simulink model "CHANGE_crazyflie_simulation_paper"  (R2019a)
settings: Solver=FixedStepAuto  StartTime=0.0  StopTime=50  FixedStep=Ts  RelTol=1e-3
values from neighbouring files (symbols this model uses):
  b = 0.033    [CHANGE_set_params_paper.m]    (also in plot_responses_paper.m = 0.25; set_params.m; set_params_paper.m)
  D_0 = 4/(Ts^2) + 4*zeta*omega_n/Ts + omega_n^2    (= 1011376)    [CHANGE_set_params_paper.m]    (also in set_params.m = 1057500; set_params_paper.m = 1057500)
  D_1 = -8/(Ts^2) + 2*omega_n^2    (= -1999872)    [CHANGE_set_params_paper.m]    (also in set_params.m = -1995000; set_params_paper.m = -1995000)
  D_2 = 4/(Ts^2) - 4*zeta*omega_n/Ts + omega_n^2    (= 988752)    [CHANGE_set_params_paper.m]    (also in set_params.m = 947500; set_params_paper.m = 947500)
  g = 9.81    [CHANGE_set_params_paper.m]    (also in set_params.m; set_params_paper.m)
  I_CF_1 = [16.823890  -1.224320  -0.716891 ... (first row only)    [CHANGE_set_params_paper.m]    (also in set_params.m; set_params_paper.m)
  I_CF_1_inv = inv(I_CF_1)    [CHANGE_set_params_paper.m]    (also in set_params.m; set_params_paper.m)
  I_rzz = 9.3e-9    (= 9.3e-09)    [CHANGE_set_params_paper.m]    (also in set_params.m; set_params_paper.m)
  k_f = 1.6e-4    (= 0.00016)    [CHANGE_set_params_paper.m]    (also in set_params.m; set_params_paper.m)
  k_m = 1e-6    (= 1e-06)    [CHANGE_set_params_paper.m]    (also in set_params.m; set_params_paper.m)
  kx = 10.25e-4    (= 0.001025)    [CHANGE_set_params_paper.m]    (also in set_params.m; set_params_paper.m)
  ky = 10.25e-4    (= 0.001025)    [CHANGE_set_params_paper.m]    (also in set_params.m; set_params_paper.m)
  kz = 7.553e-4    (= 0.0007553)    [CHANGE_set_params_paper.m]    (also in set_params.m; set_params_paper.m)
  l = 0.033    [CHANGE_set_params_paper.m]    (also in set_params.m; set_params_paper.m)
  m_CF = 0.028    [CHANGE_set_params_paper.m]    (also in set_params.m; set_params_paper.m)
  N_0 = omega_n^2    (= 64)    [CHANGE_set_params_paper.m]    (also in set_params.m = 2500; set_params_paper.m = 2500)
  N_1 = 2*omega_n^2    (= 128)    [CHANGE_set_params_paper.m]    (also in set_params.m = 5000; set_params_paper.m = 5000)
  N_2 = omega_n^2    (= 64)    [CHANGE_set_params_paper.m]    (also in set_params.m = 2500; set_params_paper.m = 2500)
  omegaR_init = [1; 1; 1; 1]*200    [CHANGE_set_params_paper.m]    (also in set_params.m; set_params_paper.m)
  T = 0.061658    [CHANGE_set_params_paper.m]    (also in inner_pd.m = 0.0666666666667; outer_pd_cs.m = 0.0666666666667; set_params.m = 0.0617; set_params_paper.m)
  T_init = m_CF*0.1    (= 0.0028)    [CHANGE_set_params_paper.m]    (also in set_params.m; set_params_paper.m)
  Ts = 1/500    (= 0.002)    [CHANGE_set_params_paper.m]    (also in inner_pd.m = 0.01; outer_pd_cs.m = 0.01; set_params.m; set_params_paper.m)
undefined symbols (not defined in the file or in its folder): DiscIntNeverNeededParam, sigbuilder_block
libraries: sharedutil x4, simulink x2
(part 2 of 2)

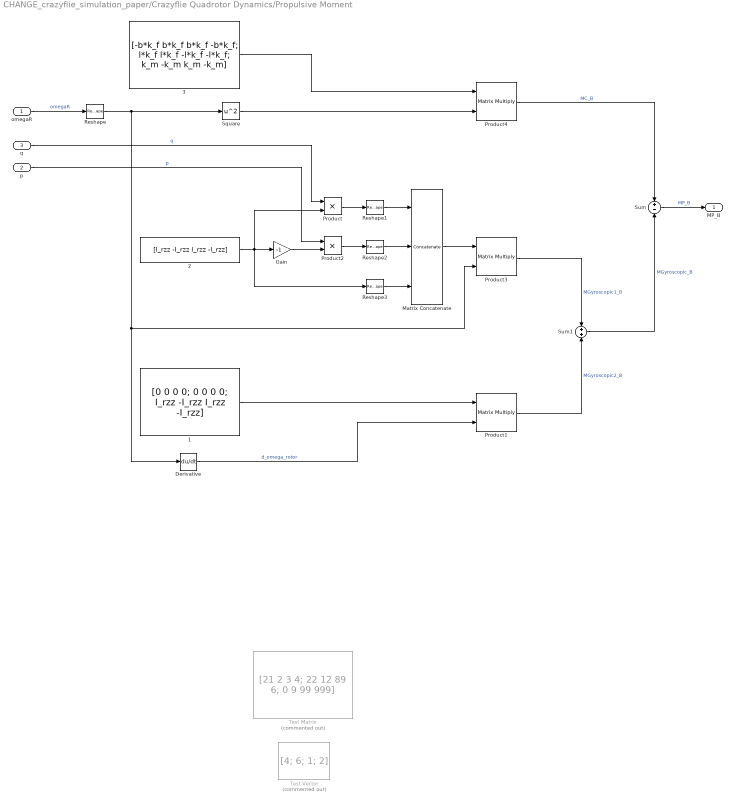
== system CHANGE_crazyflie_simulation_paper/Crazyflie Quadrotor Dynamics/Propulsive Moment ==
  omegaR : Inport
  p : Inport  Port=2
  q : Inport  Port=3
  "  1" : Constant  Value=[0 0 0 0; 0 0 0 0; I_rzz -I_rzz I_rzz -I_rzz]
  "  2" : Constant  Value=[I_rzz -I_rzz I_rzz -I_rzz]
  "  3" : Constant  Value=[-b*k_f b*k_f b*k_f -b*k_f; l*k_f l*k_f -l*k_f -l*k_f; k_m -k_m k_m -k_m]
  "  Test Matrix" : Constant  Commented=on  Value=[21 2 3 4; 22 12 89 6; 0 9 99 999]
  Derivative : Derivative
  Gain : Gain  Gain=-1
  Matrix Concatenate : Concatenate  NumInputs=3  Mode=Multidimensional array
  Product : Product
  Product1 : Product  Multiplication=Matrix(*)
  Product2 : Product
  Product3 : Product  Multiplication=Matrix(*)
  Product4 : Product  Multiplication=Matrix(*)
  Reshape : Reshape  OutputDimensionality=Column vector (2-D)
  Reshape1 : Reshape  OutputDimensionality=Row vector (2-D)
  Reshape2 : Reshape  OutputDimensionality=Row vector (2-D)
  Reshape3 : Reshape  OutputDimensionality=Row vector (2-D)
  Square : Math  Operator=square  SaturateOnIntegerOverflow=on
  Sum : Sum  Inputs=+-
  Sum1 : Sum
  Test Vector : Constant  Commented=on  Value=[4; 6; 1; 2]
  MP_B : Outport
  wires:
  Matrix Concatenate/1 -> Product3/1
  "  3"/1 -> Product4/1
  q/1 -> Product/1  "q"
  Gain/1 -> Product2/2
  Product1/1 -> Sum1/2  "MGyroscopic2_B"
  Derivative/1 -> Product1/2  "d_omega_rotor"
  "  1"/1 -> Product1/1
  Product3/1 -> Sum1/1  "MGyroscopic1_B"
  p/1 -> Product2/1  "p"
  "  2"/1 -> Product/2, Gain/1, Reshape3/1
  Product2/1 -> Reshape2/1
  Product/1 -> Reshape1/1
  Sum1/1 -> Sum/2  "MGyroscopic_B"
  Sum/1 -> MP_B/1  "MP_B"
  Product4/1 -> Sum/1  "MC_B"
  omegaR/1 -> Reshape/1  "omegaR"
  Reshape1/1 -> Matrix Concatenate/1
  Reshape2/1 -> Matrix Concatenate/2
  Reshape3/1 -> Matrix Concatenate/3
  Reshape/1 -> Square/1, Product3/2, Derivative/1
  Square/1 -> Product4/2

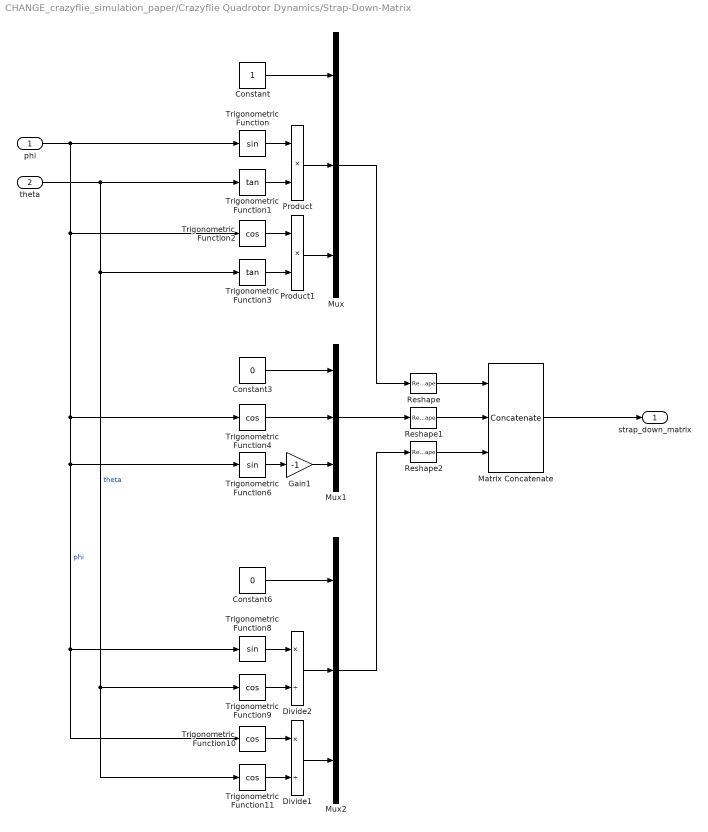
== system CHANGE_crazyflie_simulation_paper/Crazyflie Quadrotor Dynamics/Strap-Down-Matrix ==
  phi : Inport
  theta : Inport  Port=2
  Constant : Constant
  Constant3 : Constant  Value=0
  Constant6 : Constant  Value=0
  Divide1 : Product  Inputs=*/
  Divide2 : Product  Inputs=*/
  Gain1 : Gain  Gain=-1
  Matrix Concatenate : Concatenate  NumInputs=3  Mode=Multidimensional array
  Mux : Mux  Inputs=3
  Mux1 : Mux  Inputs=3
  Mux2 : Mux  Inputs=3
  Product : Product
  Product1 : Product
  Reshape : Reshape  OutputDimensionality=Row vector (2-D)
  Reshape1 : Reshape  OutputDimensionality=Row vector (2-D)
  Reshape2 : Reshape  OutputDimensionality=Row vector (2-D)
  Trigonometric Function : Trigonometry
  Trigonometric Function1 : Trigonometry  Operator=tan
  Trigonometric Function{2,4,9..11} (5 alike) : Trigonometry  Operator=cos
  Trigonometric Function3 : Trigonometry  Operator=tan
  Trigonometric Function6 : Trigonometry
  Trigonometric Function8 : Trigonometry
  strap_down_matrix : Outport
  wires:
  Gain1/1 -> Mux1/3
  Matrix Concatenate/1 -> strap_down_matrix/1
  Mux/1 -> Reshape/1
  Product1/1 -> Mux/3
  Reshape1/1 -> Matrix Concatenate/2
  Constant6/1 -> Mux2/1
  Reshape/1 -> Matrix Concatenate/1
  Constant3/1 -> Mux1/1
  Trigonometric Function4/1 -> Mux1/2
  Trigonometric Function/1 -> Product/1
  Reshape2/1 -> Matrix Concatenate/3
  theta/1 -> Trigonometric Function3/1, Trigonometric Function11/1, Trigonometric Function9/1, Trigonometric Function1/1  "theta"
  Trigonometric Function3/1 -> Product1/2
  Trigonometric Function2/1 -> Product1/1
  Product/1 -> Mux/2
  Divide1/1 -> Mux2/3
  Trigonometric Function9/1 -> Divide2/2
  Trigonometric Function6/1 -> Gain1/1
  Mux2/1 -> Reshape2/1
  Trigonometric Function8/1 -> Divide2/1
  Trigonometric Function1/1 -> Product/2
  Mux1/1 -> Reshape1/1
  Trigonometric Function10/1 -> Divide1/1
  Trigonometric Function11/1 -> Divide1/2
  Divide2/1 -> Mux2/2
  Constant/1 -> Mux/1
  phi/1 -> Trigonometric Function10/1, Trigonometric Function8/1, Trigonometric Function6/1, Trigonometric Function4/1, Trigonometric Function2/1, Trigonometric Function/1  "phi"

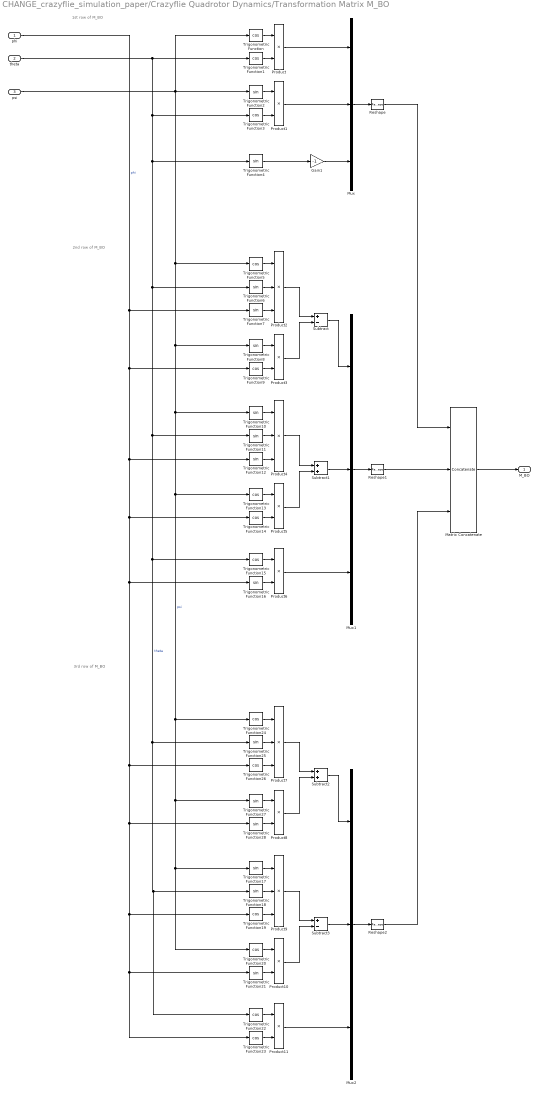
== system CHANGE_crazyflie_simulation_paper/Crazyflie Quadrotor Dynamics/Transformation Matrix M_BO ==
  note: 3rd row of M_BO
  note: 2nd row of M_BO
  note: 1st row of M_BO
  phi : Inport
  theta : Inport  Port=2
  psi : Inport  Port=3
  Gain1 : Gain  Gain=-1
  Matrix Concatenate : Concatenate  NumInputs=3  Mode=Multidimensional array
  Mux : Mux  Inputs=3
  Mux1 : Mux  Inputs=3
  Mux2 : Mux  Inputs=3
  Product{,1,3,5..6,8,10..11} (8 alike) : Product
  Product{2,4,7,9} (4 alike) : Product  Inputs=3
  Reshape : Reshape  OutputDimensionality=Row vector (2-D)
  Reshape1 : Reshape  OutputDimensionality=Row vector (2-D)
  Reshape2 : Reshape  OutputDimensionality=Row vector (2-D)
  Subtract : Sum  Inputs=+-
  Subtract1 : Sum
  Subtract2 : Sum
  Subtract3 : Sum  Inputs=+-
  Trigonometric Function{,1,3,5,9,13..15,19..20,22..24,26} (14 alike) : Trigonometry  Operator=cos
  Trigonometric Function{2,4,6..8,10..12,16..18,21,25,27..28} (15 alike) : Trigonometry
  M_BO : Outport
  wires:
  Gain1/1 -> Mux/3
  Trigonometric Function/1 -> Product/1
  Trigonometric Function1/1 -> Product/2
  psi/1 -> Trigonometric Function20/1, Trigonometric Function17/1, Trigonometric Function27/1, Trigonometric Function24/1, Trigonometric Function13/1, Trigonometric Function10/1, Trigonometric Function8/1, Trigonometric Function5/1, Trigonometric Function/1, Trigonometric Function2/1  "psi"
  Trigonometric Function3/1 -> Product1/2
  Trigonometric Function2/1 -> Product1/1
  Product/1 -> Mux/1
  Product1/1 -> Mux/2
  Trigonometric Function4/1 -> Gain1/1
  Mux/1 -> Reshape/1
  Reshape/1 -> Matrix Concatenate/1
  Trigonometric Function5/1 -> Product2/1
  Trigonometric Function6/1 -> Product2/2
  theta/1 -> Trigonometric Function22/1, Trigonometric Function18/1, Trigonometric Function25/1, Trigonometric Function15/1, Trigonometric Function11/1, Trigonometric Function6/1, Trigonometric Function4/1, Trigonometric Function3/1, Trigonometric Function1/1  "theta"
  Trigonometric Function7/1 -> Product2/3
  phi/1 -> Trigonometric Function23/1, Trigonometric Function21/1, Trigonometric Function19/1, Trigonometric Function28/1, Trigonometric Function26/1, Trigonometric Function16/1, Trigonometric Function14/1, Trigonometric Function12/1, Trigonometric Function9/1, Trigonometric Function7/1  "phi"
  Trigonometric Function8/1 -> Product3/1
  Trigonometric Function9/1 -> Product3/2
  Product2/1 -> Subtract/1
  Product3/1 -> Subtract/2
  Product5/1 -> Subtract1/2
  Product4/1 -> Subtract1/1
  Trigonometric Function14/1 -> Product5/2
  Trigonometric Function13/1 -> Product5/1
  Trigonometric Function12/1 -> Product4/3
  Trigonometric Function11/1 -> Product4/2
  Trigonometric Function10/1 -> Product4/1
  Trigonometric Function16/1 -> Product6/2
  Trigonometric Function15/1 -> Product6/1
  Subtract/1 -> Mux1/1
  Product6/1 -> Mux1/3
  Subtract1/1 -> Mux1/2
  Mux1/1 -> Reshape1/1
  Reshape1/1 -> Matrix Concatenate/2
  Reshape2/1 -> Matrix Concatenate/3
  Mux2/1 -> Reshape2/1
  Subtract3/1 -> Mux2/2
  Product11/1 -> Mux2/3
  Subtract2/1 -> Mux2/1
  Trigonometric Function22/1 -> Product11/1
  Trigonometric Function23/1 -> Product11/2
  Trigonometric Function17/1 -> Product9/1
  Trigonometric Function18/1 -> Product9/2
  Trigonometric Function19/1 -> Product9/3
  Trigonometric Function20/1 -> Product10/1
  Trigonometric Function21/1 -> Product10/2
  Product9/1 -> Subtract3/1
  Product10/1 -> Subtract3/2
  Product8/1 -> Subtract2/2
  Product7/1 -> Subtract2/1
  Trigonometric Function28/1 -> Product8/2
  Trigonometric Function27/1 -> Product8/1
  Trigonometric Function26/1 -> Product7/3
  Trigonometric Function25/1 -> Product7/2
  Trigonometric Function24/1 -> Product7/1
  Matrix Concatenate/1 -> M_BO/1

== system CHANGE_crazyflie_simulation_paper/Crazyflie Quadrotor Dynamics1/Aerodynamic Force ==
  V_B : Inport
  Demux : Demux  Outputs=3
  Gain : Gain  Gain=-kx
  Gain1 : Gain  Gain=-ky
  Gain2 : Gain  Gain=-kz
  Mux1 : Mux  Inputs=3
  Reshape : Reshape  OutputDimensionality=Column vector (2-D)
  FA_B : Outport
  wires:
  Reshape/1 -> FA_B/1  "FA_B"
  Demux/1 -> Gain/1  "v_B"
  Demux/3 -> Gain2/1  "w_B"
  V_B/1 -> Demux/1
  Demux/2 -> Gain1/1  "u_B"
  Gain/1 -> Mux1/1
  Gain1/1 -> Mux1/2
  Mux1/1 -> Reshape/1
  Gain2/1 -> Mux1/3

== system CHANGE_crazyflie_simulation_paper/Crazyflie Quadrotor Dynamics1/Cross Product Custom ==
  A : Inport
  B : Inport  Port=2
  A1 : InportShadow
  B1 : InportShadow  Port=2
  Subsystem : sharedutil/3x3 Cross Product/Subsystem  SystemSampleTime=-1
      settings: SourceProductName=Aerospace Blockset  SourceProductBaseCode=AE
  Subsystem1 : sharedutil/3x3 Cross Product/Subsystem1  SystemSampleTime=-1
      settings: SourceProductName=Aerospace Blockset  SourceProductBaseCode=AE
  Sum3 : Sum  Inputs=+|-  SaturateOnIntegerOverflow=on  InputSameDT=on  OutDataTypeStr=Inherit: Same as first input
  C : Outport
  wires:
  Subsystem/1 -> Sum3/1
  B1/1 -> Subsystem1/2
  Sum3/1 -> C/1
  B/1 -> Subsystem/2
  Subsystem1/1 -> Sum3/2
  A/1 -> Subsystem/1
  A1/1 -> Subsystem1/1

== system CHANGE_crazyflie_simulation_paper/Crazyflie Quadrotor Dynamics1/Gravitational Force  ==
  Product : Product
  Reshape : Reshape  OutputDimensionality=Column vector (2-D)
  g_acc : Constant  Value=[0; 0; g]
  m_CF : Constant  Value=m_CF
  FG_O : Outport
  wires:
  Reshape/1 -> FG_O/1  "FG_O"
  Product/1 -> Reshape/1
  g_acc/1 -> Product/1
  m_CF/1 -> Product/2

== system CHANGE_crazyflie_simulation_paper/Crazyflie Quadrotor Dynamics1/Propulsive Force ==
  omegaR : Inport
  Constant : Constant  Value=0
  Demux1 : Demux
  Gain4 : Gain  Gain=-k_f
  Matrix Sum2 : Sum  Inputs=++++
  Mux : Mux  Inputs=3
  Reshape : Reshape  OutputDimensionality=Column vector (2-D)
  FP_B : Outport
  wires:
  Constant/1 -> Mux/1, Mux/2
  Reshape/1 -> FP_B/1  "FP_B"
  Demux1/3 -> Matrix Sum2/3  "omegaR_3"
  Demux1/1 -> Matrix Sum2/1  "omegaR_1"
  Demux1/4 -> Matrix Sum2/4  "omegaR_4"
  Mux/1 -> Reshape/1
  Matrix Sum2/1 -> Gain4/1
  omegaR/1 -> Demux1/1
  Demux1/2 -> Matrix Sum2/2  "omegaR_2"
  Gain4/1 -> Mux/3

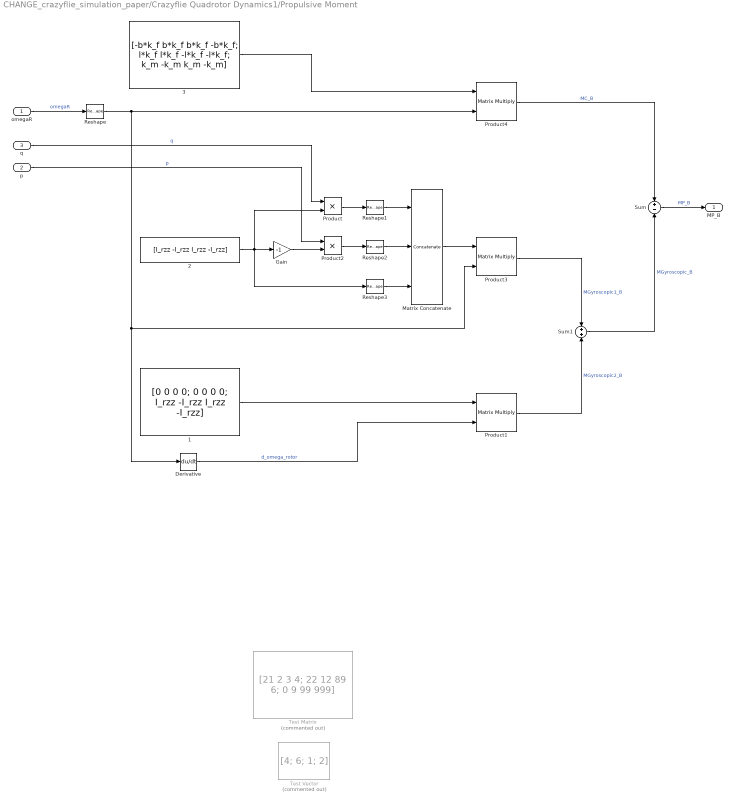
== system CHANGE_crazyflie_simulation_paper/Crazyflie Quadrotor Dynamics1/Propulsive Moment ==
  omegaR : Inport
  p : Inport  Port=2
  q : Inport  Port=3
  "  1" : Constant  Value=[0 0 0 0; 0 0 0 0; I_rzz -I_rzz I_rzz -I_rzz]
  "  2" : Constant  Value=[I_rzz -I_rzz I_rzz -I_rzz]
  "  3" : Constant  Value=[-b*k_f b*k_f b*k_f -b*k_f; l*k_f l*k_f -l*k_f -l*k_f; k_m -k_m k_m -k_m]
  "  Test Matrix" : Constant  Commented=on  Value=[21 2 3 4; 22 12 89 6; 0 9 99 999]
  Derivative : Derivative
  Gain : Gain  Gain=-1
  Matrix Concatenate : Concatenate  NumInputs=3  Mode=Multidimensional array
  Product : Product
  Product1 : Product  Multiplication=Matrix(*)
  Product2 : Product
  Product3 : Product  Multiplication=Matrix(*)
  Product4 : Product  Multiplication=Matrix(*)
  Reshape : Reshape  OutputDimensionality=Column vector (2-D)
  Reshape1 : Reshape  OutputDimensionality=Row vector (2-D)
  Reshape2 : Reshape  OutputDimensionality=Row vector (2-D)
  Reshape3 : Reshape  OutputDimensionality=Row vector (2-D)
  Sum : Sum  Inputs=+-
  Sum1 : Sum
  Test Vector : Constant  Commented=on  Value=[4; 6; 1; 2]
  MP_B : Outport
  wires:
  Matrix Concatenate/1 -> Product3/1
  "  3"/1 -> Product4/1
  Reshape/1 -> Product3/2, Derivative/1, Product4/2
  q/1 -> Product/1  "q"
  Gain/1 -> Product2/2
  Product1/1 -> Sum1/2  "MGyroscopic2_B"
  Derivative/1 -> Product1/2  "d_omega_rotor"
  "  1"/1 -> Product1/1
  Product3/1 -> Sum1/1  "MGyroscopic1_B"
  p/1 -> Product2/1  "p"
  "  2"/1 -> Product/2, Gain/1, Reshape3/1
  Product2/1 -> Reshape2/1
  Product/1 -> Reshape1/1
  Sum1/1 -> Sum/2  "MGyroscopic_B"
  Sum/1 -> MP_B/1  "MP_B"
  Product4/1 -> Sum/1  "MC_B"
  omegaR/1 -> Reshape/1  "omegaR"
  Reshape1/1 -> Matrix Concatenate/1
  Reshape2/1 -> Matrix Concatenate/2
  Reshape3/1 -> Matrix Concatenate/3

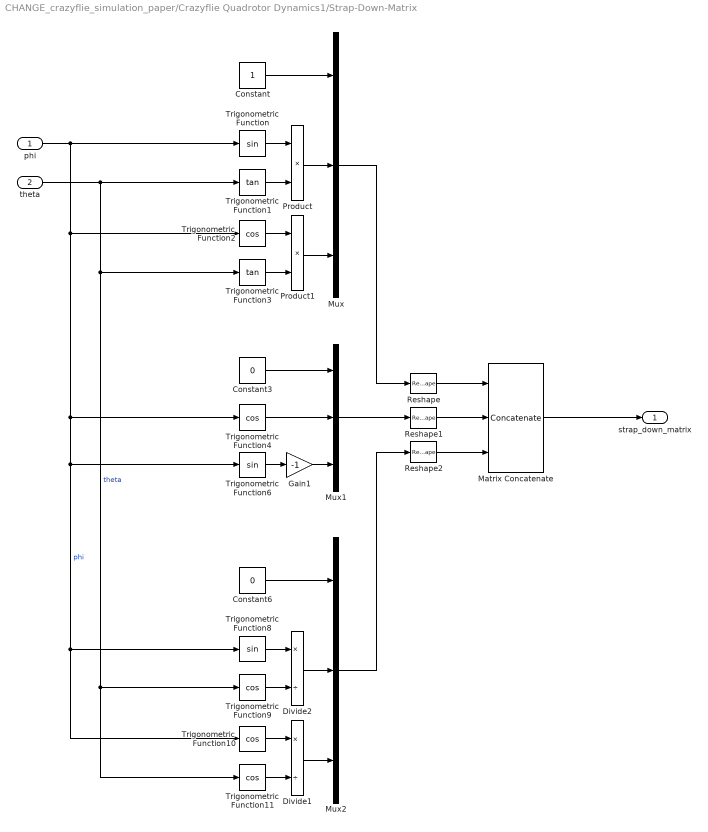
== system CHANGE_crazyflie_simulation_paper/Crazyflie Quadrotor Dynamics1/Strap-Down-Matrix ==
  phi : Inport
  theta : Inport  Port=2
  Constant : Constant
  Constant3 : Constant  Value=0
  Constant6 : Constant  Value=0
  Divide1 : Product  Inputs=*/
  Divide2 : Product  Inputs=*/
  Gain1 : Gain  Gain=-1
  Matrix Concatenate : Concatenate  NumInputs=3  Mode=Multidimensional array
  Mux : Mux  Inputs=3
  Mux1 : Mux  Inputs=3
  Mux2 : Mux  Inputs=3
  Product : Product
  Product1 : Product
  Reshape : Reshape  OutputDimensionality=Row vector (2-D)
  Reshape1 : Reshape  OutputDimensionality=Row vector (2-D)
  Reshape2 : Reshape  OutputDimensionality=Row vector (2-D)
  Trigonometric Function : Trigonometry
  Trigonometric Function1 : Trigonometry  Operator=tan
  Trigonometric Function{2,4,9..11} (5 alike) : Trigonometry  Operator=cos
  Trigonometric Function3 : Trigonometry  Operator=tan
  Trigonometric Function6 : Trigonometry
  Trigonometric Function8 : Trigonometry
  strap_down_matrix : Outport
  wires:
  Gain1/1 -> Mux1/3
  Matrix Concatenate/1 -> strap_down_matrix/1
  Mux/1 -> Reshape/1
  Product1/1 -> Mux/3
  Reshape1/1 -> Matrix Concatenate/2
  Constant6/1 -> Mux2/1
  Reshape/1 -> Matrix Concatenate/1
  Constant3/1 -> Mux1/1
  Trigonometric Function4/1 -> Mux1/2
  Trigonometric Function/1 -> Product/1
  Reshape2/1 -> Matrix Concatenate/3
  theta/1 -> Trigonometric Function3/1, Trigonometric Function11/1, Trigonometric Function9/1, Trigonometric Function1/1  "theta"
  Trigonometric Function3/1 -> Product1/2
  Trigonometric Function2/1 -> Product1/1
  Product/1 -> Mux/2
  Divide1/1 -> Mux2/3
  Trigonometric Function9/1 -> Divide2/2
  Trigonometric Function6/1 -> Gain1/1
  Mux2/1 -> Reshape2/1
  Trigonometric Function8/1 -> Divide2/1
  Trigonometric Function1/1 -> Product/2
  Mux1/1 -> Reshape1/1
  Trigonometric Function10/1 -> Divide1/1
  Trigonometric Function11/1 -> Divide1/2
  Divide2/1 -> Mux2/2
  Constant/1 -> Mux/1
  phi/1 -> Trigonometric Function10/1, Trigonometric Function8/1, Trigonometric Function6/1, Trigonometric Function4/1, Trigonometric Function2/1, Trigonometric Function/1  "phi"

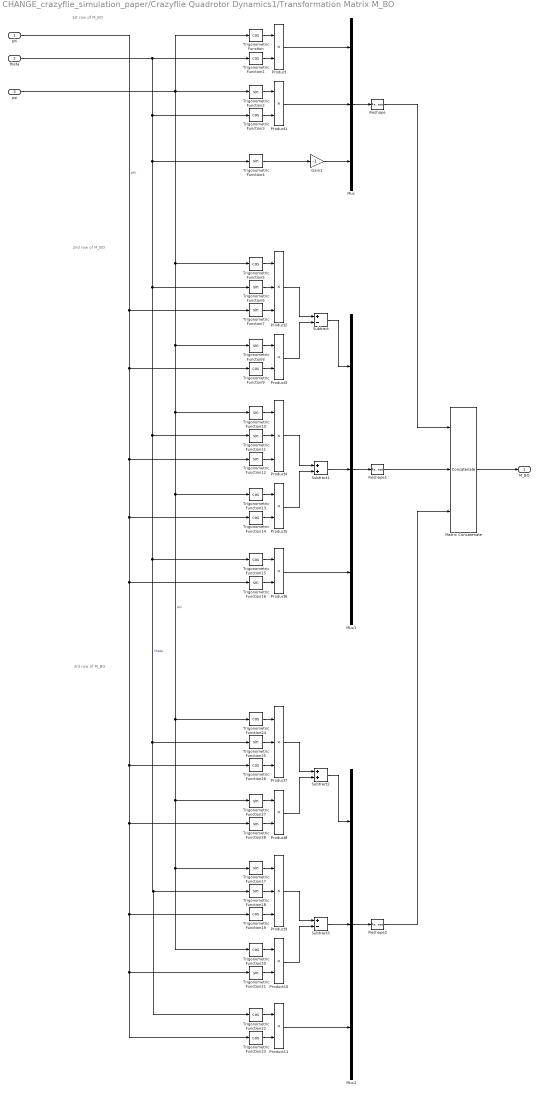
== system CHANGE_crazyflie_simulation_paper/Crazyflie Quadrotor Dynamics1/Transformation Matrix M_BO ==
  note: 3rd row of M_BO
  note: 2nd row of M_BO
  note: 1st row of M_BO
  phi : Inport
  theta : Inport  Port=2
  psi : Inport  Port=3
  Gain1 : Gain  Gain=-1
  Matrix Concatenate : Concatenate  NumInputs=3  Mode=Multidimensional array
  Mux : Mux  Inputs=3
  Mux1 : Mux  Inputs=3
  Mux2 : Mux  Inputs=3
  Product{,1,3,5..6,8,10..11} (8 alike) : Product
  Product{2,4,7,9} (4 alike) : Product  Inputs=3
  Reshape : Reshape  OutputDimensionality=Row vector (2-D)
  Reshape1 : Reshape  OutputDimensionality=Row vector (2-D)
  Reshape2 : Reshape  OutputDimensionality=Row vector (2-D)
  Subtract : Sum  Inputs=+-
  Subtract1 : Sum
  Subtract2 : Sum
  Subtract3 : Sum  Inputs=+-
  Trigonometric Function{,1,3,5,9,13..15,19..20,22..24,26} (14 alike) : Trigonometry  Operator=cos
  Trigonometric Function{2,4,6..8,10..12,16..18,21,25,27..28} (15 alike) : Trigonometry
  M_BO : Outport
  wires:
  Gain1/1 -> Mux/3
  Trigonometric Function/1 -> Product/1
  Trigonometric Function1/1 -> Product/2
  psi/1 -> Trigonometric Function20/1, Trigonometric Function17/1, Trigonometric Function27/1, Trigonometric Function24/1, Trigonometric Function13/1, Trigonometric Function10/1, Trigonometric Function8/1, Trigonometric Function5/1, Trigonometric Function/1, Trigonometric Function2/1  "psi"
  Trigonometric Function3/1 -> Product1/2
  Trigonometric Function2/1 -> Product1/1
  Product/1 -> Mux/1
  Product1/1 -> Mux/2
  Trigonometric Function4/1 -> Gain1/1
  Mux/1 -> Reshape/1
  Reshape/1 -> Matrix Concatenate/1
  Trigonometric Function5/1 -> Product2/1
  Trigonometric Function6/1 -> Product2/2
  theta/1 -> Trigonometric Function22/1, Trigonometric Function18/1, Trigonometric Function25/1, Trigonometric Function15/1, Trigonometric Function11/1, Trigonometric Function6/1, Trigonometric Function4/1, Trigonometric Function3/1, Trigonometric Function1/1  "theta"
  Trigonometric Function7/1 -> Product2/3
  phi/1 -> Trigonometric Function23/1, Trigonometric Function21/1, Trigonometric Function19/1, Trigonometric Function28/1, Trigonometric Function26/1, Trigonometric Function16/1, Trigonometric Function14/1, Trigonometric Function12/1, Trigonometric Function9/1, Trigonometric Function7/1  "phi"
  Trigonometric Function8/1 -> Product3/1
  Trigonometric Function9/1 -> Product3/2
  Product2/1 -> Subtract/1
  Product3/1 -> Subtract/2
  Product5/1 -> Subtract1/2
  Product4/1 -> Subtract1/1
  Trigonometric Function14/1 -> Product5/2
  Trigonometric Function13/1 -> Product5/1
  Trigonometric Function12/1 -> Product4/3
  Trigonometric Function11/1 -> Product4/2
  Trigonometric Function10/1 -> Product4/1
  Trigonometric Function16/1 -> Product6/2
  Trigonometric Function15/1 -> Product6/1
  Subtract/1 -> Mux1/1
  Product6/1 -> Mux1/3
  Subtract1/1 -> Mux1/2
  Mux1/1 -> Reshape1/1
  Reshape1/1 -> Matrix Concatenate/2
  Reshape2/1 -> Matrix Concatenate/3
  Mux2/1 -> Reshape2/1
  Subtract3/1 -> Mux2/2
  Product11/1 -> Mux2/3
  Subtract2/1 -> Mux2/1
  Trigonometric Function22/1 -> Product11/1
  Trigonometric Function23/1 -> Product11/2
  Trigonometric Function17/1 -> Product9/1
  Trigonometric Function18/1 -> Product9/2
  Trigonometric Function19/1 -> Product9/3
  Trigonometric Function20/1 -> Product10/1
  Trigonometric Function21/1 -> Product10/2
  Product9/1 -> Subtract3/1
  Product10/1 -> Subtract3/2
  Product8/1 -> Subtract2/2
  Product7/1 -> Subtract2/1
  Trigonometric Function28/1 -> Product8/2
  Trigonometric Function27/1 -> Product8/1
  Trigonometric Function26/1 -> Product7/3
  Trigonometric Function25/1 -> Product7/2
  Trigonometric Function24/1 -> Product7/1
  Matrix Concatenate/1 -> M_BO/1

== matlab function CHANGE_crazyflie_simulation_paper/Pseudoinverse of u  ==
  data: u input; y output size=[3 3]
function y = fcn(u)

y = pinv(u);

== matlab function CHANGE_crazyflie_simulation_paper/Pseudoinverse of u ==
  data: u input; y output
function y = fcn(u)

y = pinv(u);

== matlab function CHANGE_crazyflie_simulation_paper/Pseudoinverse of u 1 ==
  data: u input; y output size=[3 3]
function y = fcn(u)

y = pinv(u);

== matlab function CHANGE_crazyflie_simulation_paper/Pseudoinverse of u1 ==
  data: u input; y output
function y = fcn(u)

y = pinv(u);
